simulink model "mtrmodel_bozuculu"  (R2020b)
settings: Solver=VariableStepAuto  StartTime=0.0  StopTime=8  RelTol=1e-3
values from neighbouring files (symbols this model uses):
  Ki = (kv*T)/gz    [PID Katsayilari.m]
  T = 0.0325    [PID Katsayilari.m]
undefined symbols (not defined in the file or in its folder): Be, Je, Kb, kd, ki, kp, La, Ra
settings Model: Creator=HCS  LastModifiedBy=HCS

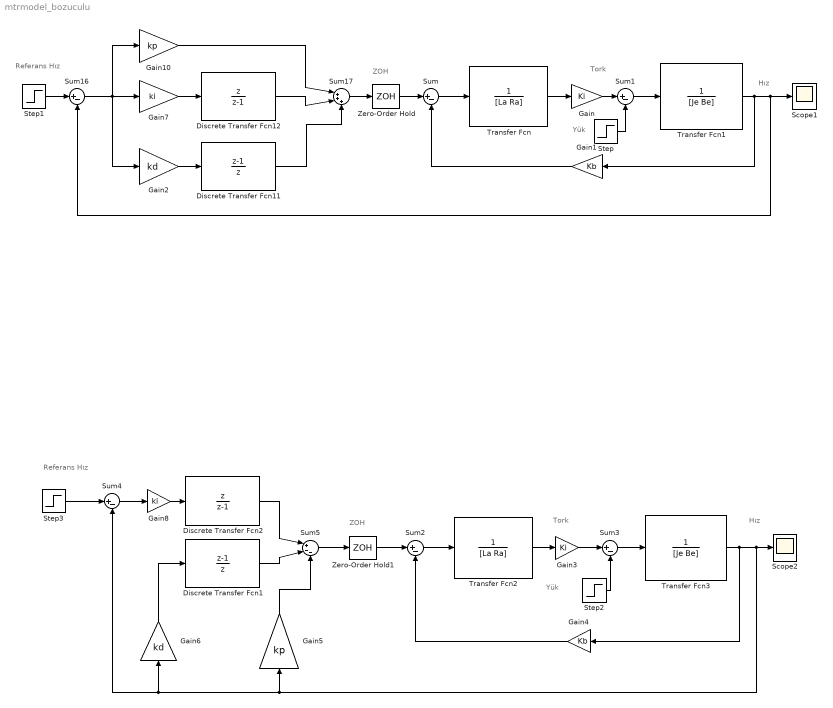
== system mtrmodel_bozuculu ==
  note: Referans Hız
  note: ZOH
  note: Hız
  note: Tork
  note: Yük
  note: Hız
  note: Tork
  note: Yük
  note: ZOH
  note: Referans Hız
  Discrete Transfer Fcn1 : DiscreteTransferFcn  Numerator=[1 -1]  Denominator=[1 0]
  Discrete Transfer Fcn11 : DiscreteTransferFcn  Numerator=[1 -1]  Denominator=[1 0]
  Discrete Transfer Fcn12 : DiscreteTransferFcn  Numerator=[1 0]  Denominator=[1 -1]
  Discrete Transfer Fcn2 : DiscreteTransferFcn  Numerator=[1 0]  Denominator=[1 -1]
  Gain : Gain  Gain=Ki
  Gain1 : Gain  Gain=Kb
  Gain10 : Gain  Gain=kp
  Gain2 : Gain  Gain=kd
  Gain3 : Gain  Gain=Ki
  Gain4 : Gain  Gain=Kb
  Gain5 : Gain  Gain=kp
  Gain6 : Gain  Gain=kd
  Gain7 : Gain  Gain=ki
  Gain8 : Gain  Gain=ki
  Scope1 : Scope
  Scope2 : Scope
  Step{,1..3} (4 alike) : Step  SampleTime=0
  Sum{,1..4,16} (6 alike) : Sum  Inputs=|+-
  Sum17 : Sum  Inputs=|+++
  Sum5 : Sum  Inputs=|+--
  Transfer Fcn : TransferFcn  Denominator=[La Ra]
  Transfer Fcn1 : TransferFcn  Denominator=[Je Be]
  Transfer Fcn2 : TransferFcn  Denominator=[La Ra]
  Transfer Fcn3 : TransferFcn  Denominator=[Je Be]
  Zero-Order Hold : ZeroOrderHold  SampleTime=T
  Zero-Order Hold1 : ZeroOrderHold  SampleTime=T
  wires:
  Step1/1 -> Sum16/1
  Discrete Transfer Fcn11/1 -> Sum17/3
  Gain2/1 -> Discrete Transfer Fcn11/1
  Gain7/1 -> Discrete Transfer Fcn12/1
  Gain10/1 -> Sum17/1
  Discrete Transfer Fcn12/1 -> Sum17/2
  Sum16/1 -> Gain2/1, Gain10/1, Gain7/1
  Sum17/1 -> Zero-Order Hold/1
  Sum/1 -> Transfer Fcn/1
  Transfer Fcn/1 -> Gain/1
  Zero-Order Hold/1 -> Sum/1
  Gain1/1 -> Sum/2
  Transfer Fcn1/1 -> Scope1/1, Sum16/2, Gain1/1
  Gain/1 -> Sum1/1
  Sum1/1 -> Transfer Fcn1/1
  Zero-Order Hold1/1 -> Sum2/1
  Step3/1 -> Sum4/1
  Sum3/1 -> Transfer Fcn3/1
  Gain3/1 -> Sum3/1
  Gain8/1 -> Discrete Transfer Fcn2/1
  Sum4/1 -> Gain8/1
  Transfer Fcn2/1 -> Gain3/1
  Discrete Transfer Fcn2/1 -> Sum5/1
  Gain6/1 -> Discrete Transfer Fcn1/1
  Gain4/1 -> Sum2/2
  Sum2/1 -> Transfer Fcn2/1
  Sum5/1 -> Zero-Order Hold1/1
  Gain5/1 -> Sum5/3
  Transfer Fcn3/1 -> Scope2/1, Sum4/2, Gain6/1, Gain5/1, Gain4/1
  Step/1 -> Sum1/2
  Discrete Transfer Fcn1/1 -> Sum5/2
  Step2/1 -> Sum3/2
